simulink model "Pendulum_Stabilizer"  (R2013a)
settings: Solver=ode45  StartTime=0.0  StopTime=10.0  RelTol=1e-3
undefined symbols (not defined in the file or in its folder): K_mat
settings Model: Creator=s4357594  LastModifiedBy=s4357594

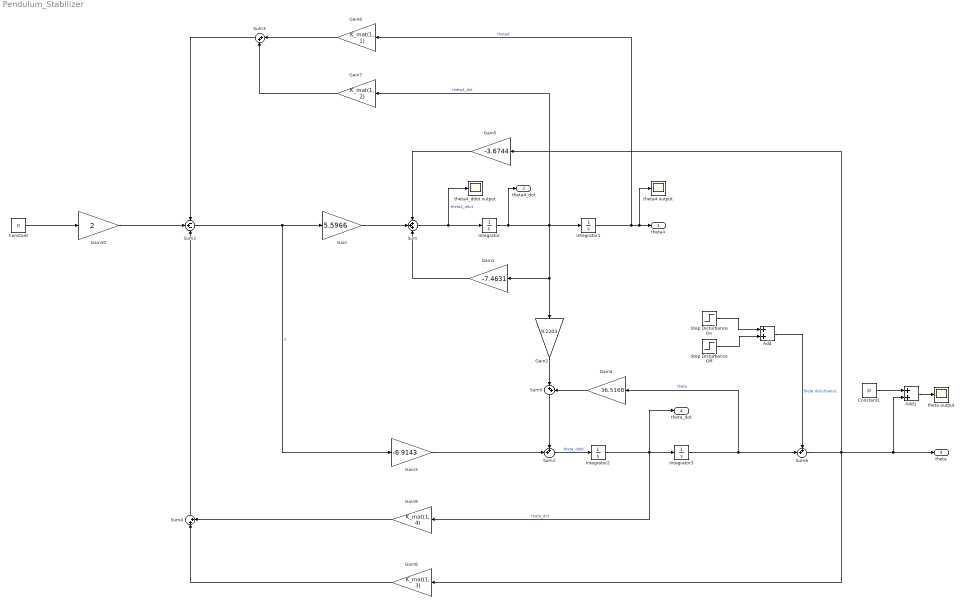
== system Pendulum_Stabilizer ==
  Add : Sum
  Add1 : Sum
  Constant : Constant  Value=0
  Constant1 : Constant  Value=pi
  Gain : Gain  Gain=5.5966
  Gain1 : Gain  Gain=-7.4631
  Gain10 : Gain  Gain=2
  Gain2 : Gain  Gain=9.2203
  Gain3 : Gain  Gain=-6.9143
  Gain4 : Gain  Gain=36.5168
  Gain5 : Gain  Gain=-3.6744
  Gain6 : Gain  Gain=K_mat(1, 1)
  Gain7 : Gain  Gain=K_mat(1, 2)
  Gain8 : Gain  Gain=K_mat(1, 3)
  Gain9 : Gain  Gain=K_mat(1, 4)
  Integrator{,1..3} (4 alike) : Integrator
  Step Disturbance Off : Step  Time=1.025  After=-0.1  SampleTime=0
  Step Disturbance On : Step  After=0.1  SampleTime=0
  Sum : Sum  Inputs=+++
  Sum1 : Sum  Inputs=++|
  Sum2 : Sum  Inputs=-+-
  Sum3 : Sum  Inputs=|++
  Sum4 : Sum  Inputs=|++
  Sum5 : Sum  Inputs=|++
  Sum6 : Sum  Inputs=++|
  theta output : Scope
  theta4 output : Scope
  theta4_ddot output : Scope
      settings: SaveName=ScopeData2
  theta4 : Outport
  theta4_dot : Outport  Port=2
  theta : Outport  Port=3
  theta_dot : Outport  Port=4
  wires:
  Sum2/1 -> Gain3/1, Gain/1  "u"
  Gain/1 -> Sum/2
  Sum/1 -> theta4_ddot output/1, Integrator/1  "theta4_ddot"
  Integrator/1 -> theta4_dot/1, Gain7/1, Integrator1/1, Gain1/1, Gain2/1  "theta4_dot"
  Integrator1/1 -> Gain6/1, theta4 output/1, theta4/1  "theta4"
  Gain1/1 -> Sum/3
  Gain5/1 -> Sum/1
  Gain2/1 -> Sum5/1
  Gain3/1 -> Sum1/2
  Sum1/1 -> Integrator2/1  "theta_ddot"
  Integrator2/1 -> theta_dot/1, Gain9/1, Integrator3/1  "theta_dot"
  Gain6/1 -> Sum3/1
  Gain7/1 -> Sum3/2
  Gain8/1 -> Sum4/1
  Gain9/1 -> Sum4/2
  Gain4/1 -> Sum5/2
  Sum5/1 -> Sum1/1
  Constant/1 -> Gain10/1
  Sum4/1 -> Sum2/3
  Sum3/1 -> Sum2/1
  Gain10/1 -> Sum2/2
  Step Disturbance On/1 -> Add/1
  Step Disturbance Off/1 -> Add/2
  Integrator3/1 -> Gain4/1, Sum6/2  "theta"
  Add/1 -> Sum6/1  "theta disturbance"
  Sum6/1 -> Gain8/1, Gain5/1, Add1/2, theta/1
  Constant1/1 -> Add1/1
  Add1/1 -> theta output/1
